simulink model "SCIM13"  (R2016a)
settings: Solver=FixedStepAuto  StartTime=0.0  StopTime=5  FixedStep=0.0001  RelTol=1e-3
values from neighbouring files (symbols this model uses):
  Lm = 0.1271    [motor4_workspace.mat]    (also in motor_wrapper.m = obj.Lm; scim_verifier.m = obj.motor.getLm(); setMotorParams.m; stationary_class.m = obj.Lm)
  Lr = 0.2744    [motor4_workspace.mat]    (also in motor_wrapper.m = obj.Lr; scim_verifier.m = obj.motor.getLr(); setMotorParams.m; stationary_class.m = obj.Lr)
  Ls = 0.2744    [motor4_workspace.mat]    (also in motor_wrapper.m = obj.Ls; scim_verifier.m = obj.motor.getLs(); setMotorParams.m; stationary.m = Ls/10)
  M_ab02abc = [1  0  1; -0.5  0.866025403784  1; -0.5  -0.866025403784  1]    [motor4_workspace.mat]    (also in setMotorParams.m = inv(M_abc2ab0); workspaceSav.mat)
  M_abc2ab0 = [0.666666666667  -0.333333333333  -0.333333333333; 0  0.57735026919  -0.57735026919; 0.333333333333  0.333333333333  0.333333333333]    [motor4_workspace.mat]    (also in setMotorParams.m = 2/3*[1, -0.5, -0.5; 0, sqrt(3)/2, -sqrt(3)/2;  0.5, 0.5, 0.5; workspaceSav.mat)
  Rr = 1.009    [motor4_workspace.mat]    (also in motor_wrapper.m = obj.Rr; setMotorParams.m; stationary_class.m = obj.Rr; stationary_from_eq.m = obj.Rr)
  sig = (tox-fromx)/6    [gaussSpace.m]    (also in motor4_workspace.mat = 0.785452782217; setMotorParams.m = 0.785452782217; stationary_class.m = 1-Lm*Lm/Ls/Lr; torqueFinder.m = 0.785452782217)
libraries: simulink x2, powerlib_meascontrol x1
settings Model: Creator=ebenera  LastModifiedBy=ebenera

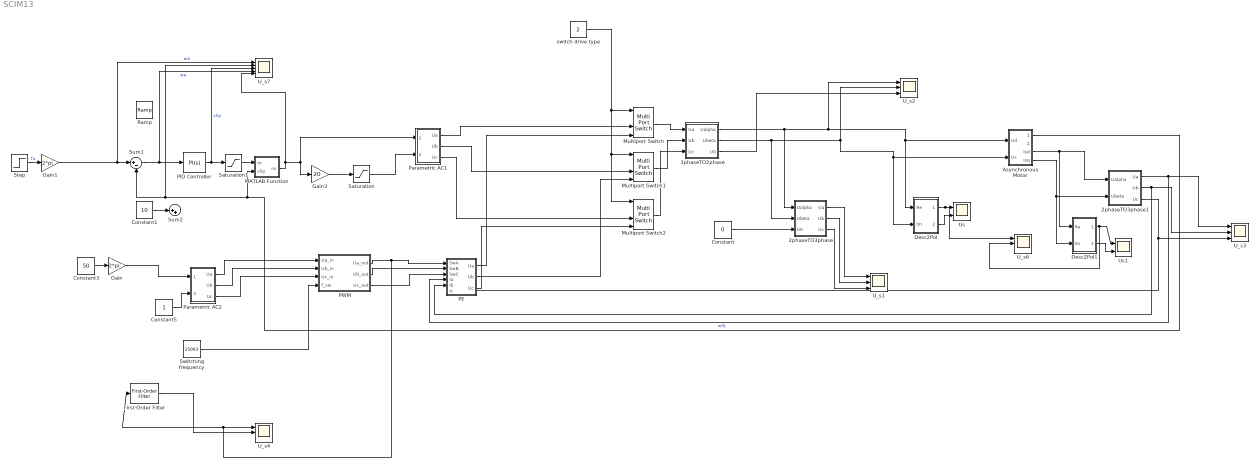
== system SCIM13 ==
  2phaseTO3phase : Subsystem
  2phaseTO3phase1 : Subsystem
  "3phaseTO2phase " : Subsystem
  Asynchronous Motor : Subsystem
  Constant : Constant  Value=0
  Constant1 : Constant  Value=10
  Constant3 : Constant  Value=50
  Constant5 : Constant
  Desc2Pol : Subsystem
  Desc2Pol1 : Subsystem
  First-Order Filter : powerlib_meascontrol/Filters/First-Order Filter  FilterType=Lowpass  Tc=1/400  Ts=0  Initialize=on  Vac_Init=[0, 0, 60]  Vdc_Init=0  PlotResponse=off  FreqRange="[0,  200,  1]"
  Gain : Gain  Gain=2*pi
  Gain1 : Gain  Gain=2*pi
  Gain3 : Gain  Gain=20
  MATLAB Function : MATLAB Function  TreatAsAtomicUnit=on
  Multiport Switch : MultiPortSwitch
  Multiport Switch1 : MultiPortSwitch
  Multiport Switch2 : MultiPortSwitch
  PE : Subsystem
  PID Controller : simulink/Continuous/PID Controller  Controller=PI  TimeDomain=Continuous-time  SampleTime=-1  IntegratorMethod=Forward Euler  FilterMethod=Forward Euler  Form=Ideal  UseFilter=on  ControllerParametersSource=internal  P=8  I=0.01  D=0  N=100  InitialConditionSource=internal  InitialConditionForIntegrator=0  InitialConditionForFilter=0  ExternalReset=none  LimitOutput=off  UpperSaturationLimit=inf  LowerSaturationLimit=-inf  LinearizeAsGain=on  AntiWindupMode=none  Kb=1  TrackingMode=off  Kt=1  PParamMin=[]  PParamMax=[]  IParamMin=[]  IParamMax=[]  DParamMin=[]  DParamMax=[]  NParamMin=[]  NParamMax=[]  KbParamMin=[]  KbParamMax=[]  KtParamMin=[]  KtParamMax=[]  POutMin=[]  POutMax=[]  IOutMin=[]  IOutMax=[]  DOutMin=[]  DOutMax=[]  NOutMin=[]  NOutMax=[]  KbOutMin=[]  KbOutMax=[]  KtOutMin=[]  KtOutMax=[]  IntegratorOutMin=[]  IntegratorOutMax=[]  FilterOutMin=[]  FilterOutMax=[]  SumOutMin=[]  SumOutMax=[]  SumI1OutMin=[]  SumI1OutMax=[]  SumI2OutMin=[]  SumI2OutMax=[]  SumI3OutMin=[]  SumI3OutMax=[]  SumDOutMin=[]  SumDOutMax=[]  SaturationOutMin=[]  SaturationOutMax=[]  IntegratorContinuousStateAttributes=''  IntegratorStateMustResolveToSignalObject=off  IntegratorRTWStateStorageClass=Auto  FilterContinuousStateAttributes=''  FilterStateMustResolveToSignalObject=off  FilterRTWStateStorageClass=Auto  DifferentiatorICPrevScaledInput=0  DifferentiatorOutMin=[]  DifferentiatorOutMax=[]
  PWM : Subsystem
  Parametric AC1 : Subsystem
  Parametric AC2 : Subsystem  Description=Generates a 3 phase supply with the given angular speed, and aplitude.
  Ramp : simulink/Sources/Ramp  slope=5  start=0  X0=1
  Saturation : Saturate  UpperLimit=300  LowerLimit=50
  Saturation1 : Saturate  UpperLimit=100  LowerLimit=-100
  Step : Step  Time=0.5  After=50  SampleTime=0
  Sum1 : Sum  Inputs=|+-
  Sum2 : Sum  Inputs=|++
  Switching frequency : Constant  Value=15003
  U_s{1..4,6} (5 alike) : Scope  NumInputPorts=3
  U_s7 : Scope  NumInputPorts=5
  Us : Scope  NumInputPorts=2
  Us1 : Scope  NumInputPorts=2
  switch drive type : Constant  Value=2
  wires:
  "3phaseTO2phase "/1(Ualpha) -> 2phaseTO3phase/1(Ualpha), U_s2/1, Desc2Pol/1(Re), Asynchronous Motor/1(Ud)
  "3phaseTO2phase "/2(Ubeta) -> 2phaseTO3phase/2(Ubeta), Asynchronous Motor/2(Us), Desc2Pol/2(Im), U_s2/2
  Desc2Pol/1(Amp) -> U_s6/1, Us/1
  Desc2Pol/2(Angle) -> Us/2
  "3phaseTO2phase "/3(U0) -> U_s2/3
  Constant/1 -> 2phaseTO3phase/3(U0)
  2phaseTO3phase/1(Ua) -> U_s1/1
  2phaseTO3phase/2(Ub) -> U_s1/2
  2phaseTO3phase/3(Uc) -> U_s1/3
  2phaseTO3phase1/1(Ua) -> PE/4(Ia), U_s3/1
  2phaseTO3phase1/2(Ub) -> PE/5(Ib), U_s3/2
  2phaseTO3phase1/3(Uc) -> PE/6(Ic), U_s3/3
  Multiport Switch/1 -> "3phaseTO2phase "/1(Ua)
  Multiport Switch1/1 -> "3phaseTO2phase "/2(Ub)
  Multiport Switch2/1 -> "3phaseTO2phase "/3(Uc)
  Parametric AC1/1(Ua) -> Multiport Switch/3
  Parametric AC1/2(Ub) -> Multiport Switch1/3
  Parametric AC1/3(Uc) -> Multiport Switch2/3
  PE/1(Ua) -> Multiport Switch/4
  PE/2(Ub) -> Multiport Switch1/4
  PE/3(Uc) -> Multiport Switch2/4
  switch drive type/1 -> Multiport Switch2/1, Multiport Switch1/1, Multiport Switch/1
  Asynchronous Motor/1(Omega) -> U_s7/2, Sum1/2, MATLAB Function/2(slip)  "wfb"
  Constant1/1 -> Sum2/1
  PWM/1(Ua_out) -> U_s4/1, First-Order Filter/1, PE/1(SwA)
  PWM/2(Ub_out) -> PE/2(SwB)
  PWM/3(Uc_out) -> PE/3(SwC)
  Parametric AC2/1(Ua) -> PWM/1(Ua_in)
  Gain/1 -> Parametric AC2/1(Omega)
  Constant5/1 -> Parametric AC2/2(Amp)
  First-Order Filter/1 -> U_s4/2
  Switching frequency/1 -> PWM/4(f_sw)
  Parametric AC2/2(Ub) -> PWM/2(Ub_in)
  Parametric AC2/3(Uc) -> PWM/3(Uc_in)
  MATLAB Function/1(ns) -> Parametric AC1/1(Omega), Gain3/1, U_s7/5
  PID Controller/1 -> Saturation1/1, U_s7/3  "slip"
  Constant3/1 -> Gain/1
  Gain3/1 -> Saturation/1
  Saturation/1 -> Parametric AC1/2(Amp)
  Asynchronous Motor/3(Isd) -> 2phaseTO3phase1/1(Ualpha), Desc2Pol1/1(Re)
  Asynchronous Motor/4(Isq) -> Desc2Pol1/2(Im), 2phaseTO3phase1/2(Ubeta)
  Desc2Pol1/1(Amp) -> U_s6/2, Us1/1
  Desc2Pol1/2(Angle) -> Us1/2
  Gain1/1 -> U_s7/1, Sum1/1  "wa"
  Sum1/1 -> U_s7/4, PID Controller/1  "we"
  Saturation1/1 -> MATLAB Function/1(nr)
  Step/1 -> Gain1/1  "fa"

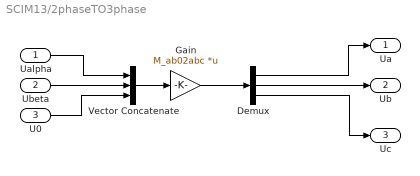
== system SCIM13/2phaseTO3phase ==
  Ualpha : Inport
  Ubeta : Inport  Port=2
  U0 : Inport  Port=3
  Demux : Demux  Outputs=3
  Gain : Gain  Gain=M_ab02abc  Multiplication=Matrix(K*u)
  Vector Concatenate : Concatenate  NumInputs=3
  Ua : Outport
  Ub : Outport  Port=2
  Uc : Outport  Port=3
  wires:
  Vector Concatenate/1 -> Gain/1
  Ualpha/1 -> Vector Concatenate/1
  Demux/3 -> Uc/1
  Gain/1 -> Demux/1
  U0/1 -> Vector Concatenate/3
  Ubeta/1 -> Vector Concatenate/2
  Demux/1 -> Ua/1
  Demux/2 -> Ub/1

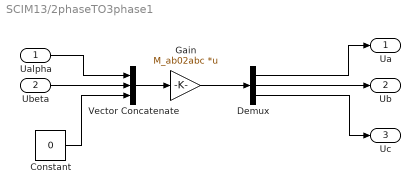
== system SCIM13/2phaseTO3phase1 ==
  Ualpha : Inport
  Ubeta : Inport  Port=2
  Constant : Constant  Value=0
  Demux : Demux  Outputs=3
  Gain : Gain  Gain=M_ab02abc  Multiplication=Matrix(K*u)
  Vector Concatenate : Concatenate  NumInputs=3
  Ua : Outport
  Ub : Outport  Port=2
  Uc : Outport  Port=3
  wires:
  Vector Concatenate/1 -> Gain/1
  Ualpha/1 -> Vector Concatenate/1
  Demux/3 -> Uc/1
  Gain/1 -> Demux/1
  Constant/1 -> Vector Concatenate/3
  Ubeta/1 -> Vector Concatenate/2
  Demux/1 -> Ua/1
  Demux/2 -> Ub/1

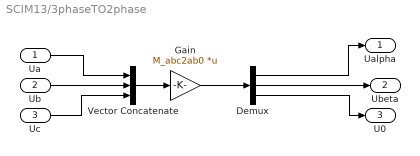
== system SCIM13/3phaseTO2phase  ==
  Ua : Inport
  Ub : Inport  Port=2
  Uc : Inport  Port=3
  Demux : Demux  Outputs=3
  Gain : Gain  Gain=M_abc2ab0  Multiplication=Matrix(K*u)
  Vector Concatenate : Concatenate  NumInputs=3
  Ualpha : Outport
  Ubeta : Outport  Port=2
  U0 : Outport  Port=3
  wires:
  Vector Concatenate/1 -> Gain/1
  Ua/1 -> Vector Concatenate/1
  Demux/3 -> U0/1
  Gain/1 -> Demux/1
  Uc/1 -> Vector Concatenate/3
  Ub/1 -> Vector Concatenate/2
  Demux/1 -> Ualpha/1
  Demux/2 -> Ubeta/1

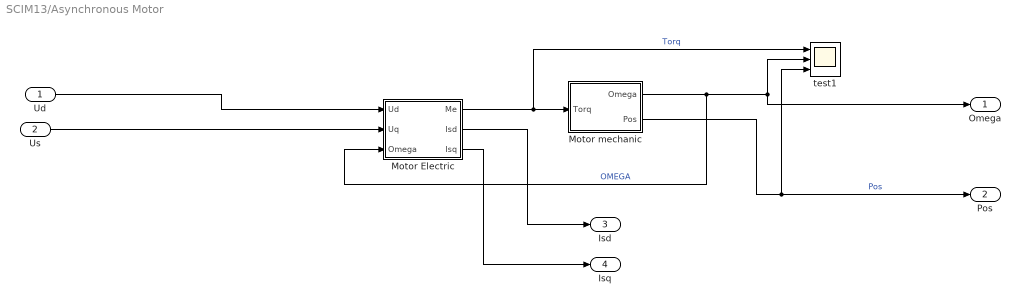
== system SCIM13/Asynchronous Motor ==
  Ud : Inport
  Us : Inport  Port=2
  Motor Electric : Subsystem
  Motor mechanic : Subsystem
  test1 : Scope  NumInputPorts=3
  Omega : Outport
  Pos : Outport  Port=2
  Isd : Outport  Port=3
  Isq : Outport  Port=4
  wires:
  Motor mechanic/2(Pos) -> test1/3, Pos/1  "Pos"
  Motor mechanic/1(Omega) -> test1/2, Omega/1, Motor Electric/3(Omega)  "OMEGA"
  Motor Electric/1(Me) -> test1/1, Motor mechanic/1("Torq ")  "Torq"
  Motor Electric/2(Isd) -> Isd/1
  Motor Electric/3(Isq) -> Isq/1
  Us/1 -> Motor Electric/2(Uq)
  Ud/1 -> Motor Electric/1(Ud)

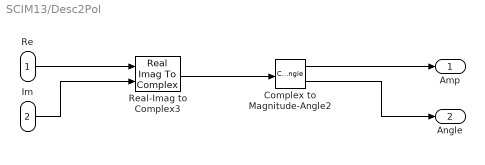
== system SCIM13/Desc2Pol ==
  Re : Inport
  Im : Inport  Port=2
  Complex to Magnitude-Angle2 : ComplexToMagnitudeAngle
  Real-Imag to Complex3 : RealImagToComplex
  Amp : Outport
  Angle : Outport  Port=2
  wires:
  Complex to Magnitude-Angle2/1 -> Amp/1
  Real-Imag to Complex3/1 -> Complex to Magnitude-Angle2/1
  Complex to Magnitude-Angle2/2 -> Angle/1
  Re/1 -> Real-Imag to Complex3/1
  Im/1 -> Real-Imag to Complex3/2

== system SCIM13/Desc2Pol1 ==
  Re : Inport
  Im : Inport  Port=2
  Complex to Magnitude-Angle2 : ComplexToMagnitudeAngle
  Real-Imag to Complex3 : RealImagToComplex
  Amp : Outport
  Angle : Outport  Port=2
  wires:
  Complex to Magnitude-Angle2/1 -> Amp/1
  Real-Imag to Complex3/1 -> Complex to Magnitude-Angle2/1
  Complex to Magnitude-Angle2/2 -> Angle/1
  Re/1 -> Real-Imag to Complex3/1
  Im/1 -> Real-Imag to Complex3/2

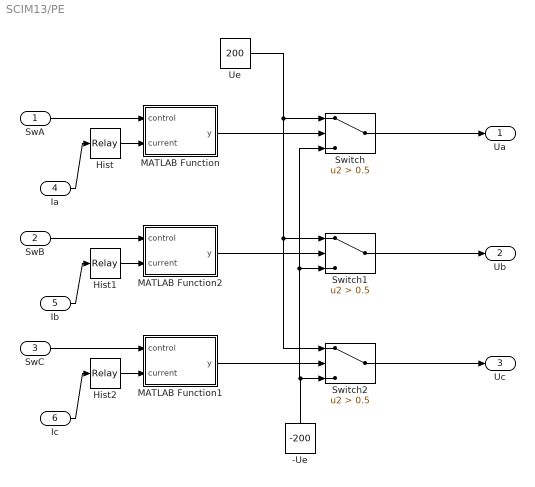
== system SCIM13/PE ==
  SwA : Inport
  SwB : Inport  Port=2
  SwC : Inport  Port=3
  Ia : Inport  Port=4
  Ib : Inport  Port=5
  Ic : Inport  Port=6
  -Ue : Constant  Value=-200
  Hist : Relay  OnSwitchValue=0.1  OffSwitchValue=-0.5  OffOutputValue=-1
  Hist1 : Relay  OnSwitchValue=0.1  OffSwitchValue=-0.5  OffOutputValue=-1
  Hist2 : Relay  OnSwitchValue=0.1  OffSwitchValue=-0.5  OffOutputValue=-1
  MATLAB Function : MATLAB Function  TreatAsAtomicUnit=on
  MATLAB Function1 : MATLAB Function  TreatAsAtomicUnit=on
  MATLAB Function2 : MATLAB Function  TreatAsAtomicUnit=on
  Switch : Switch  Criteria=u2 > Threshold  Threshold=0.5
  Switch1 : Switch  Criteria=u2 > Threshold  Threshold=0.5
  Switch2 : Switch  Criteria=u2 > Threshold  Threshold=0.5
  Ue : Constant  Value=200
  Ua : Outport
  Ub : Outport  Port=2
  Uc : Outport  Port=3
  wires:
  -Ue/1 -> Switch/3, Switch1/3, Switch2/3
  Switch/1 -> Ua/1
  Ue/1 -> Switch2/1, Switch1/1, Switch/1
  Switch1/1 -> Ub/1
  Switch2/1 -> Uc/1
  MATLAB Function/1(y) -> Switch/2
  MATLAB Function2/1(y) -> Switch1/2
  MATLAB Function1/1(y) -> Switch2/2
  SwB/1 -> MATLAB Function2/1(control)
  SwA/1 -> MATLAB Function/1(control)
  SwC/1 -> MATLAB Function1/1(control)
  Ia/1 -> Hist/1
  Hist/1 -> MATLAB Function/2(current)
  Ib/1 -> Hist1/1
  Hist1/1 -> MATLAB Function2/2(current)
  Hist2/1 -> MATLAB Function1/2(current)
  Ic/1 -> Hist2/1

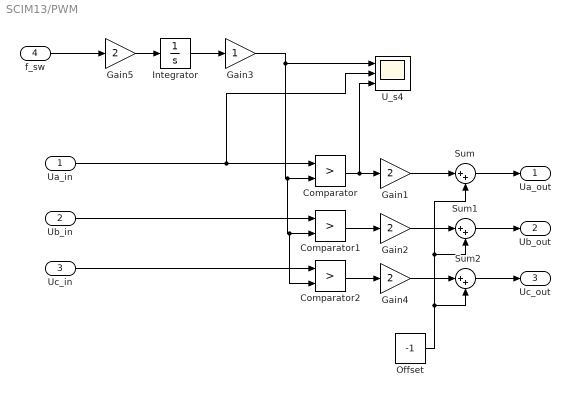
== system SCIM13/PWM ==
  Ua_in : Inport
  Ub_in : Inport  Port=2
  Uc_in : Inport  Port=3
  f_sw : Inport  Port=4
  Comparator : RelationalOperator  Operator=>  OutDataTypeStr=boolean
  Comparator1 : RelationalOperator  Operator=>  OutDataTypeStr=boolean
  Comparator2 : RelationalOperator  Operator=>  OutDataTypeStr=boolean
  Gain{1..2,4..5} (4 alike) : Gain  Gain=2
  Gain3 : Gain
  Integrator : Integrator  WrapState=on  WrappedStateUpperValue=1.01  WrappedStateLowerValue=-1.01
  Offset : Constant  Value=-1
  Sum : Sum  Inputs=|++
  Sum1 : Sum  Inputs=|++
  Sum2 : Sum  Inputs=|++
  U_s4 : Scope  NumInputPorts=3
  Ua_out : Outport
  Ub_out : Outport  Port=2
  Uc_out : Outport  Port=3
  wires:
  Uc_in/1 -> Comparator2/1
  Ub_in/1 -> Comparator1/1
  Ua_in/1 -> U_s4/2, Comparator/1
  Comparator/1 -> Gain1/1, U_s4/3
  Integrator/1 -> Gain3/1
  Gain3/1 -> U_s4/1, Comparator2/2, Comparator1/2, Comparator/2
  Gain2/1 -> Sum1/1
  Comparator1/1 -> Gain2/1
  Comparator2/1 -> Gain4/1
  Gain4/1 -> Sum2/1
  Sum2/1 -> Uc_out/1
  Sum1/1 -> Ub_out/1
  Sum/1 -> Ua_out/1
  Gain1/1 -> Sum/1
  Offset/1 -> Sum2/2, Sum1/2, Sum/2
  Gain5/1 -> Integrator/1
  f_sw/1 -> Gain5/1

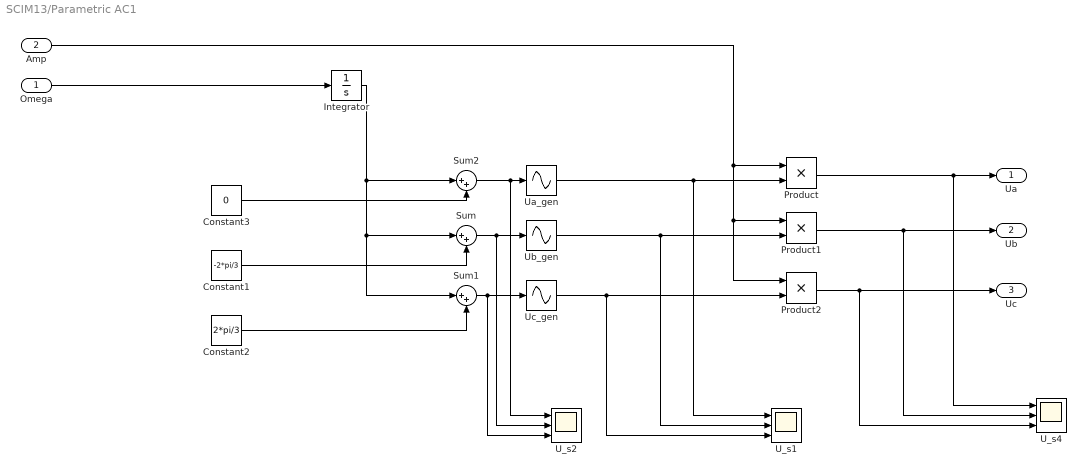
== system SCIM13/Parametric AC1 ==
  Omega : Inport
  Amp : Inport  Port=2
  Constant1 : Constant  Value=-2*pi/3
  Constant2 : Constant  Value=2*pi/3
  Constant3 : Constant  Value=0
  Integrator : Integrator  WrapState=on
  Product : Product
  Product1 : Product
  Product2 : Product
  Sum : Sum  Inputs=|++
  Sum1 : Sum  Inputs=|++
  Sum2 : Sum  Inputs=|++
  U_s1 : Scope  NumInputPorts=3
  U_s2 : Scope  NumInputPorts=3
  U_s4 : Scope  NumInputPorts=3
  Ua_gen : Sin  TimeSource=Use external signal  SampleTime=0
  Ub_gen : Sin  TimeSource=Use external signal  SampleTime=0
  Uc_gen : Sin  TimeSource=Use external signal  SampleTime=0
  Ua : Outport
  Ub : Outport  Port=2
  Uc : Outport  Port=3
  wires:
  Sum/1 -> U_s2/2, Ub_gen/1
  Omega/1 -> Integrator/1
  Constant1/1 -> Sum/2
  Constant2/1 -> Sum1/2
  Sum1/1 -> U_s2/3, Uc_gen/1
  Sum2/1 -> U_s2/1, Ua_gen/1
  Constant3/1 -> Sum2/2
  Integrator/1 -> Sum2/1, Sum1/1, Sum/1
  Product/1 -> U_s4/1, Ua/1
  Product2/1 -> U_s4/3, Uc/1
  Product1/1 -> U_s4/2, Ub/1
  Amp/1 -> Product/1, Product1/1, Product2/1
  Ua_gen/1 -> U_s1/1, Product/2
  Uc_gen/1 -> U_s1/3, Product2/2
  Ub_gen/1 -> U_s1/2, Product1/2

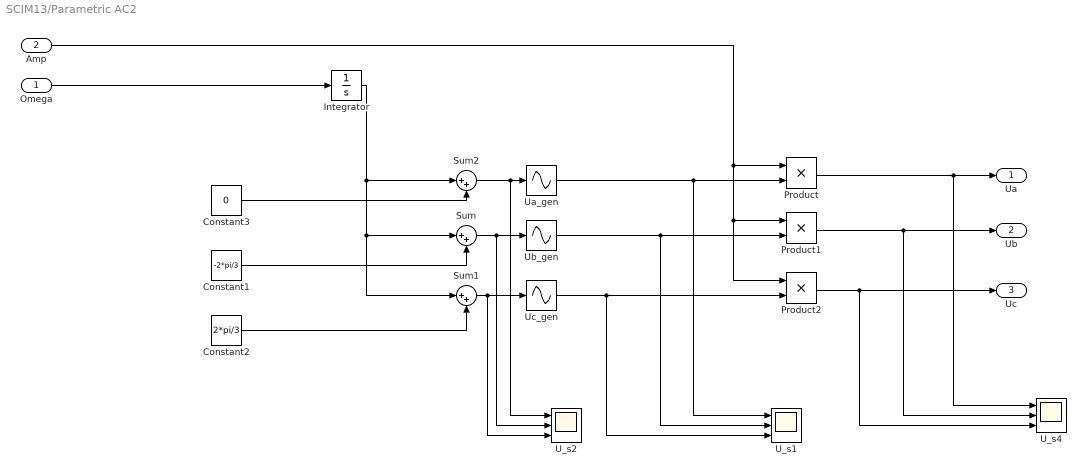
== system SCIM13/Parametric AC2 ==
  Omega : Inport
  Amp : Inport  Port=2
  Constant1 : Constant  Value=-2*pi/3
  Constant2 : Constant  Value=2*pi/3
  Constant3 : Constant  Value=0
  Integrator : Integrator  WrapState=on
  Product : Product
  Product1 : Product
  Product2 : Product
  Sum : Sum  Inputs=|++
  Sum1 : Sum  Inputs=|++
  Sum2 : Sum  Inputs=|++
  U_s1 : Scope  NumInputPorts=3
  U_s2 : Scope  NumInputPorts=3
  U_s4 : Scope  NumInputPorts=3
  Ua_gen : Sin  TimeSource=Use external signal  SampleTime=0
  Ub_gen : Sin  TimeSource=Use external signal  SampleTime=0
  Uc_gen : Sin  TimeSource=Use external signal  SampleTime=0
  Ua : Outport
  Ub : Outport  Port=2
  Uc : Outport  Port=3
  wires:
  Sum/1 -> U_s2/2, Ub_gen/1
  Omega/1 -> Integrator/1
  Constant1/1 -> Sum/2
  Constant2/1 -> Sum1/2
  Sum1/1 -> U_s2/3, Uc_gen/1
  Sum2/1 -> U_s2/1, Ua_gen/1
  Constant3/1 -> Sum2/2
  Integrator/1 -> Sum2/1, Sum1/1, Sum/1
  Product/1 -> U_s4/1, Ua/1
  Product2/1 -> U_s4/3, Uc/1
  Product1/1 -> U_s4/2, Ub/1
  Amp/1 -> Product/1, Product1/1, Product2/1
  Ua_gen/1 -> U_s1/1, Product/2
  Uc_gen/1 -> U_s1/3, Product2/2
  Ub_gen/1 -> U_s1/2, Product1/2

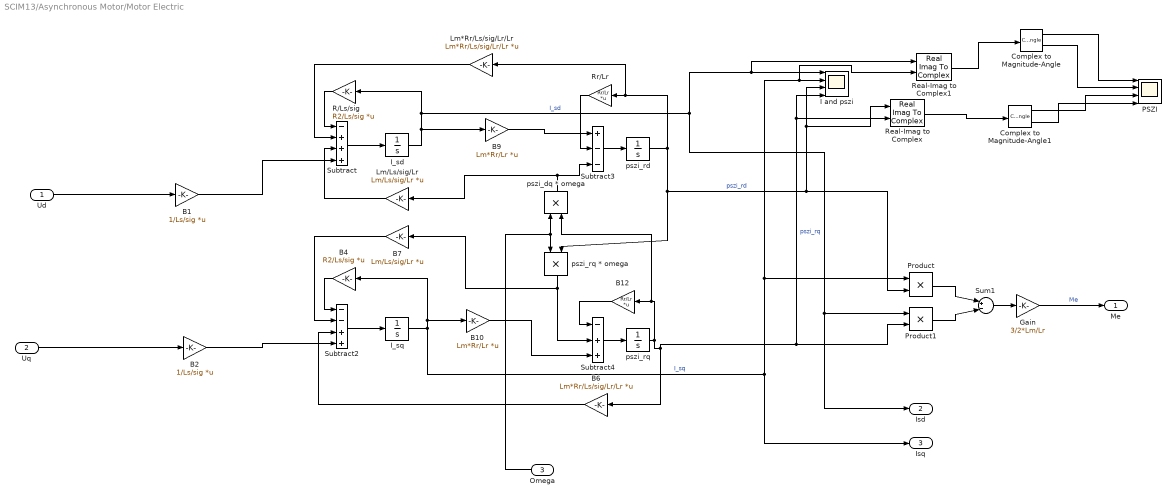
== system SCIM13/Asynchronous Motor/Motor Electric ==
  Ud : Inport
  Uq : Inport  Port=2
  Omega : Inport  Port=3
  B1 : Gain  Gain=1/Ls/sig  Multiplication=Matrix(K*u)
  B10 : Gain  Gain=Lm*Rr/Lr  Multiplication=Matrix(K*u)
  B12 : Gain  Gain=Rr/Lr  Multiplication=Matrix(K*u)
  B2 : Gain  Gain=1/Ls/sig  Multiplication=Matrix(K*u)
  B4 : Gain  Gain=R2/Ls/sig  Multiplication=Matrix(K*u)
  B6 : Gain  Gain=Lm*Rr/Ls/sig/Lr/Lr  Multiplication=Matrix(K*u)
  B7 : Gain  Gain=Lm/Ls/sig/Lr  Multiplication=Matrix(K*u)
  B9 : Gain  Gain=Lm*Rr/Lr  Multiplication=Matrix(K*u)
  Complex to Magnitude-Angle : ComplexToMagnitudeAngle
  Complex to Magnitude-Angle1 : ComplexToMagnitudeAngle
  Gain : Gain  Gain=3/2*Lm/Lr
  I and pszi : Scope  NumInputPorts=4
  I_sd : Integrator
  I_sq : Integrator
  Lm*Rr/Ls/sig/Lr/Lr : Gain  Gain=Lm*Rr/Ls/sig/Lr/Lr  Multiplication=Matrix(K*u)
  Lm/Ls/sig/Lr : Gain  Gain=Lm/Ls/sig/Lr  Multiplication=Matrix(K*u)
  PSZI : Scope  NumInputPorts=4
  Product : Product
  Product1 : Product
  R/Ls/sig : Gain  Gain=R2/Ls/sig  Multiplication=Matrix(K*u)
  Real-Imag to Complex : RealImagToComplex
  Real-Imag to Complex1 : RealImagToComplex
  Rr/Lr : Gain  Gain=Rr/Lr  Multiplication=Matrix(K*u)
  Subtract : Sum  Inputs=-+++
  Subtract2 : Sum  Inputs=--++
  Subtract3 : Sum  Inputs=+--
  Subtract4 : Sum  Inputs=-++
  Sum1 : Sum  Inputs=|+-|
  pszi_dq * omega : Product
  pszi_rd : Integrator
  "pszi_rq " : Integrator
  pszi_rq * omega : Product
  Me : Outport
  Isd : Outport  Port=2
  Isq : Outport  Port=3
  wires:
  pszi_rq * omega/1 -> Subtract4/2, B7/1
  Subtract/1 -> I_sd/1
  B12/1 -> Subtract4/1
  Product1/1 -> Sum1/2
  Lm*Rr/Ls/sig/Lr/Lr/1 -> Subtract/2
  Product/1 -> Sum1/1
  I_sq/1 -> Isq/1, Real-Imag to Complex1/2, I and pszi/2, Product/1, B10/1, B4/1  "I_sq"
  I_sd/1 -> B9/1, Isd/1, Product1/1, Real-Imag to Complex1/1, I and pszi/1, R/Ls/sig/1  "I_sd"
  Sum1/1 -> Gain/1
  R/Ls/sig/1 -> Subtract/1
  B6/1 -> Subtract2/3
  B4/1 -> Subtract2/1
  pszi_dq * omega/1 -> Subtract3/3, Lm/Ls/sig/Lr/1
  Omega/1 -> pszi_rq * omega/1, pszi_dq * omega/1
  B9/1 -> Subtract3/1
  Rr/Lr/1 -> Subtract3/2
  pszi_rd/1 -> Real-Imag to Complex/1, I and pszi/3, Product/2, pszi_rq * omega/2, Lm*Rr/Ls/sig/Lr/Lr/1, Rr/Lr/1  "pszi_rd"
  Lm/Ls/sig/Lr/1 -> Subtract/3
  "pszi_rq "/1 -> pszi_dq * omega/2, B12/1, Real-Imag to Complex/2, I and pszi/4, Product1/2, B6/1  "pszi_rq"
  B7/1 -> Subtract2/2
  Gain/1 -> Me/1  "Me"
  B10/1 -> Subtract4/3
  Subtract4/1 -> "pszi_rq "/1
  Subtract2/1 -> I_sq/1
  Subtract3/1 -> pszi_rd/1
  Uq/1 -> B2/1
  Ud/1 -> B1/1
  B1/1 -> Subtract/4
  B2/1 -> Subtract2/4
  Real-Imag to Complex1/1 -> Complex to Magnitude-Angle/1
  Complex to Magnitude-Angle/1 -> PSZI/1
  Complex to Magnitude-Angle/2 -> PSZI/2
  Real-Imag to Complex/1 -> Complex to Magnitude-Angle1/1
  Complex to Magnitude-Angle1/1 -> PSZI/3
  Complex to Magnitude-Angle1/2 -> PSZI/4

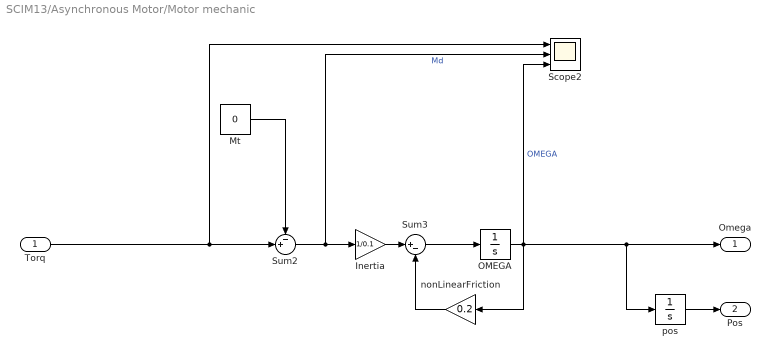
== system SCIM13/Asynchronous Motor/Motor mechanic ==
  "Torq " : Inport
  Inertia : Gain  Gain=1/0.1
  Mt : Constant  Value=0
  OMEGA : Integrator
  Scope2 : Scope  NumInputPorts=3
  Sum2 : Sum  Inputs=-+|
  Sum3 : Sum  Inputs=|+-
  nonLinearFriction : Gain  Gain=0.2
  pos : Integrator  WrapState=on
  Omega : Outport
  Pos : Outport  Port=2
  wires:
  "Torq "/1 -> Scope2/1, Sum2/2
  OMEGA/1 -> Scope2/3, pos/1, Omega/1, nonLinearFriction/1  "OMEGA"
  Sum3/1 -> OMEGA/1
  Sum2/1 -> Inertia/1, Scope2/2  "Md"
  Mt/1 -> Sum2/1
  nonLinearFriction/1 -> Sum3/2
  Inertia/1 -> Sum3/1
  pos/1 -> Pos/1

== matlab function SCIM13/PE/MATLAB Function1 ==
  data: control input; y output; current input
function y = fcn(control, current)
	if control >= 1
        y = 1;
    elseif control <= -1
        y=-1;
    elseif(current>0)
        y = -1;
    else
        y = 1;
    end
end

== matlab function SCIM13/PE/MATLAB Function ==
  data: control input; y output; current input
function y = fcn(control, current)
	if control >= 1
        y = 1;
    elseif control <= -1
        y=-1;
    elseif(current>0)
        y = -1;
    else
        y = 1;
    end
end

== matlab function SCIM13/PE/MATLAB Function2 ==
  data: control input; y output; current input
function y = fcn(control, current)
	if control >= 1
        y = 1;
    elseif control <= -1
        y=-1;
    elseif(current>0)
        y = -1;
    else
        y = 1;
    end
end

== matlab function SCIM13/MATLAB Function ==
  data: nr input; ns output; slip input
function ns = fcn(nr, slip)
    ns = nr/(1-slip);
end
